simulink model "V_F_Control_induction_motor"  (R2017a)
settings: Solver=ode23t  StartTime=0.0  StopTime=10  FixedStep=1e-6  RelTol=1e-3
libraries: powerlib x10, simulink x3
settings Model: SimulationMode=accelerator  Creator=Aslam  LastModifiedBy=Administrator
settings DataIOCC: SaveFormat=StructureWithTime
settings OptimizationCC: LifeSpan=inf
settings DebuggingCC: SFExecutionAtInitializationDiag=none
settings HardwareCC: ProdBitPerSizeT=32  ProdBitPerPtrDiffT=32  ProdWordSize=32  ProdHWDeviceType=Specified

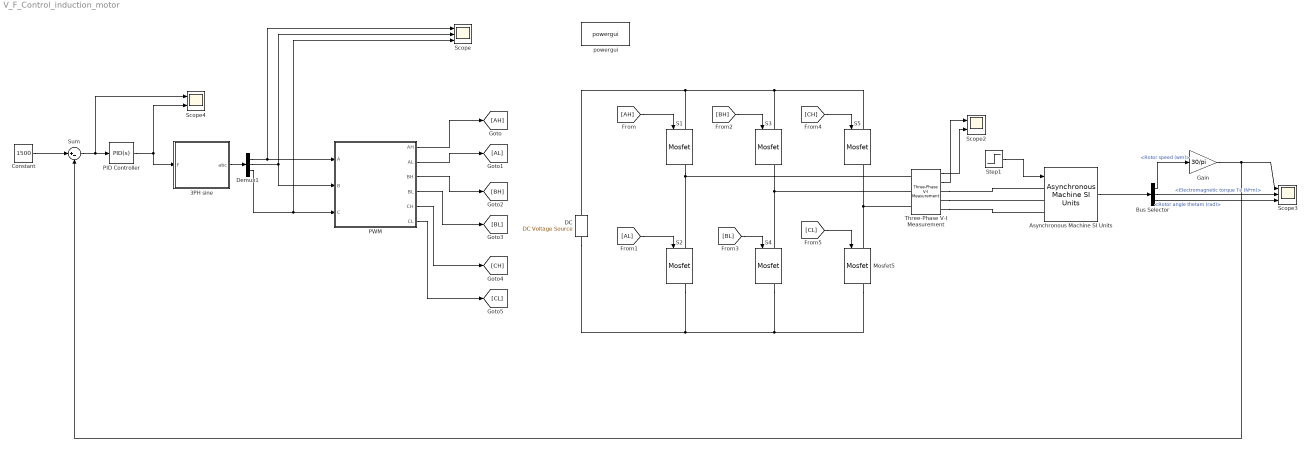
== system V_F_Control_induction_motor ==
  3PH sine : Subsystem
  Asynchronous Machine SI Units : powerlib/Machines/Asynchronous Machine SI Units  RotorType=Squirrel-cage  PresetModel="01:  5 HP   460 V 60Hz 1750 RPM"  MechanicalLoad=Torque Tm  ShowDetailedParameters=on  ReferenceFrame=Rotor  Units=SI  MeasurementBus=off  NominalParameters=[3730 460 60]  Stator=[1.115 0.005974]  Rotor=[1.083 0.005974]  Cage1=[0.4155 0.002066]  Cage2=[0.4168 0.0003495]  Lm=0.2037  Mechanical=[0.02 0.005752 2]  PolePairs=2  InitialConditions=[0 0 0 0 0 0 0 0]  SimulateSaturation=off  Saturation=[14.03593122, 27.81365428, 53.79336849, 72.68890987, 97.98006896, 148.6815601, 215.7428561, 302.9841135, 428.7778367 ; 230, 322, 414, 460, 506, 552, 598, 644, 690]  LoadFlowParameters=1492000  TsPowergui=0  TsBlock=-1  IterativeModel=Trapezoidal non iterative  IterativeDiscreteModel=Trapezoidal non iterative  Pmec=1.492e+006
  Bus Selector : BusSelector  OutputSignals=Mechanical.Rotor speed (wm),Mechanical.Electromagnetic torque Te (N*m),Mechanical.Rotor angle thetam (rad)
  Constant : Constant  Value=1500
  DC : powerlib/Electrical Sources/DC Voltage Source  Amplitude=600  Measurements=None
  Demux1 : Demux  Outputs=3
  Gain : Gain  Gain=30/pi
  Mosfet5 : powerlib/Power Electronics/Mosfet  Ron=0.1  Lon=0  Rd=0.01  Vfd=0  IC=0  Rs=1e5  Cs=inf  Measurements=on
  PID Controller : simulink/Continuous/PID Controller  Controller=PID  TimeDomain=Continuous-time  SampleTime=-1  IntegratorMethod=Forward Euler  FilterMethod=Forward Euler  Form=Parallel  UseFilter=on  ControllerParametersSource=internal  P=0.01  I=0.1  D=0  N=100  InitialConditionSource=internal  InitialConditionForIntegrator=0  InitialConditionForFilter=0  ExternalReset=none  LimitOutput=off  UpperSaturationLimit=inf  LowerSaturationLimit=-inf  LinearizeAsGain=on  AntiWindupMode=none  Kb=1  TrackingMode=off  Kt=1  PParamMin=[]  PParamMax=[]  IParamMin=[]  IParamMax=[]  DParamMin=[]  DParamMax=[]  NParamMin=[]  NParamMax=[]  KbParamMin=[]  KbParamMax=[]  KtParamMin=[]  KtParamMax=[]  POutMin=[]  POutMax=[]  IOutMin=[]  IOutMax=[]  DOutMin=[]  DOutMax=[]  NOutMin=[]  NOutMax=[]  KbOutMin=[]  KbOutMax=[]  KtOutMin=[]  KtOutMax=[]  IntegratorOutMin=[]  IntegratorOutMax=[]  FilterOutMin=[]  FilterOutMax=[]  SumOutMin=[]  SumOutMax=[]  SumI1OutMin=[]  SumI1OutMax=[]  SumI2OutMin=[]  SumI2OutMax=[]  SumI3OutMin=[]  SumI3OutMax=[]  SumDOutMin=[]  SumDOutMax=[]  SaturationOutMin=[]  SaturationOutMax=[]  IntegratorContinuousStateAttributes=''  IntegratorStateMustResolveToSignalObject=off  IntegratorRTWStateStorageClass=Auto  FilterContinuousStateAttributes=''  FilterStateMustResolveToSignalObject=off  FilterRTWStateStorageClass=Auto  DifferentiatorICPrevScaledInput=0  DifferentiatorOutMin=[]  DifferentiatorOutMax=[]  InitialConditionSetting=State (most efficient)
  PWM : Subsystem
  S{1..5} (5 alike) : powerlib/Power Electronics/Mosfet  Ron=0.1  Lon=0  Rd=0.01  Vfd=0  IC=0  Rs=1e5  Cs=inf  Measurements=on
  Scope : Scope  NumInputPorts=3
  Scope2 : Scope  NumInputPorts=2
  Scope3 : Scope  NumInputPorts=3
  Scope4 : Scope  NumInputPorts=2
  Step1 : Step  Time=5  Before=5  After=10  SampleTime=0
  Sum : Sum  Inputs=|+-
  Three-Phase V-I Measurement : powerlib/Measurements/Three-Phase V-I Measurement  VoltageMeasurement=phase-to-phase  SetLabelV=off  LabelV=Vabc  Vpu=off  VpuLL=off  CurrentMeasurement=yes  SetLabelI=off  LabelI=Iabc  Ipu=off  Pbase=100e6  Vbase=500e3  OutputType=Complex  PhasorSimulation=off  PSBequivalent=0
  powergui : powerlib/powergui  Priority=1  SimulationMode=Discrete  SampleTime=10e-6  frequency=60  Iterations=50  frequencyindice=0  Pbase=100e6  ErrMax=1e-4  UnitsV=kV  UnitsW=MW  buscounter=0  FunctionMessages=off  echomessages=off  EnableUseOfTLC=off  CurrentSourceSwitches=off  DisableSnubberDevices=off  DisableRonSwitches=off  DisableVfSwitches=off  DisplayEquations=off  SolverType=Tustin/Backward Euler (TBE)  Interpol=off  ExternalGateDelay=off  methode=off  Ts=100  x0status=blocks  SPID=off  SwTol=0  HookPort=off  RestoreLinks=warning  ResistiveCurrentMeasurement=off  Frange=[0:2:500]  Ylog=off  Xlog=on  ShowGrid=off  save=off  variable=ZData  structure=0  ZoomFFT=off  StartTime=0.0  cycles=1  DisplayStyle=1  fundamental=60  FreqAxis=off  MaxFrequency=1000  frequencyindicesteady=1  RmsSteady=1  display=off
  wires:
  Demux1/1 -> Scope/1, PWM/1(A)
  Demux1/2 -> Scope/2, PWM/2(B)
  Demux1/3 -> Scope/3, PWM/3(C)
  PWM/1(AH) -> [AH]
  PWM/2(AL) -> [AL]
  PWM/3(BH) -> [BH]
  PWM/4(BL) -> [BL]
  PWM/5(CH) -> [CH]
  PWM/6(CL) -> [CL]
  [AH] -> S1/1
  [AL] -> S2/1
  [BH] -> S3/1
  [BL] -> S4/1
  [CH] -> S5/1
  [CL] -> Mosfet5/1
  Three-Phase V-I Measurement/2 -> Scope2/1
  Three-Phase V-I Measurement/1 -> Scope2/2
  Asynchronous Machine SI Units/1 -> Bus Selector/1
  Bus Selector/1 -> Gain/1  "<Rotor speed (wm)>"
  Bus Selector/2 -> Scope3/2  "<Electromagnetic torque Te (N*m)>"
  Bus Selector/3 -> Scope3/3  "<Rotor angle thetam (rad)>"
  Gain/1 -> Sum/2, Scope3/1
  Sum/1 -> Scope4/1, PID Controller/1
  Constant/1 -> Sum/1
  PID Controller/1 -> 3PH sine/1(F), Scope4/2
  3PH sine/1(abc) -> Demux1/1
  Step1/1 -> Asynchronous Machine SI Units/1
  connections:
  DC/RConn1 -- S5/LConn1 -- S3/LConn1 -- S1/LConn1
  DC/LConn1 -- S2/RConn1 -- Mosfet5/RConn1 -- S4/RConn1
  Mosfet5/LConn1 -- Three-Phase V-I Measurement/LConn3 -- S5/RConn1
  S4/LConn1 -- Three-Phase V-I Measurement/LConn2 -- S3/RConn1
  S1/RConn1 -- S2/LConn1 -- Three-Phase V-I Measurement/LConn1
  Three-Phase V-I Measurement/RConn1 -- Asynchronous Machine SI Units/LConn1
  Three-Phase V-I Measurement/RConn2 -- Asynchronous Machine SI Units/LConn2
  Three-Phase V-I Measurement/RConn3 -- Asynchronous Machine SI Units/LConn3

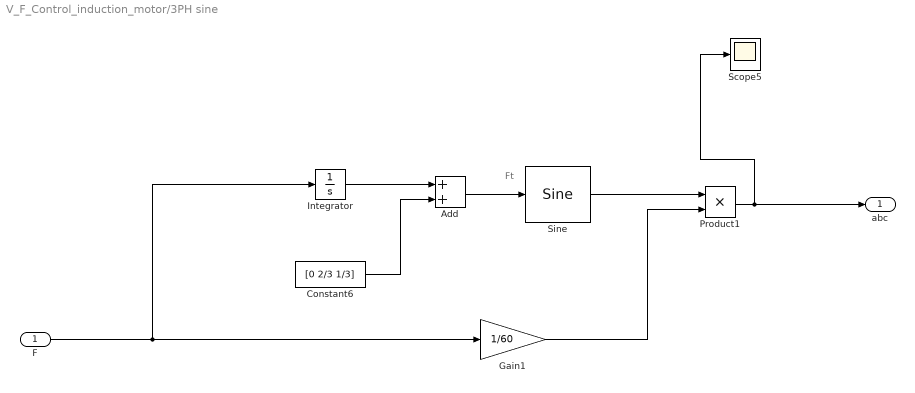
== system V_F_Control_induction_motor/3PH sine ==
  note: Ft
  F : Inport
  Add : Sum
  Constant6 : Constant  Value=[0 2/3 1/3]
  Gain1 : Gain  Gain=1/60
  Integrator : Integrator
  Product1 : Product
  Scope5 : Scope
  Sine : simulink/Lookup Tables/Sine  Formula=sin(2*pi*u)  NumDataPoints=(2^5)+1  OutputWordLength=16  InternalRulePriority=Speed
      settings: SourceProductName=Simulink
  abc : Outport
  wires:
  F/1 -> Gain1/1, Integrator/1
  Gain1/1 -> Product1/2
  Sine/1 -> Product1/1
  Product1/1 -> abc/1, Scope5/1
  Constant6/1 -> Add/2
  Add/1 -> Sine/1
  Integrator/1 -> Add/1

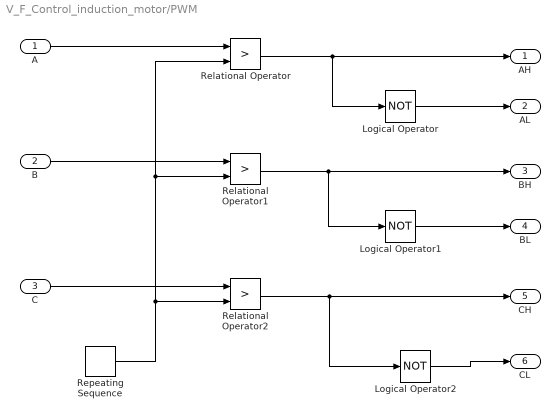
== system V_F_Control_induction_motor/PWM ==
  A : Inport
  B : Inport  Port=2
  C : Inport  Port=3
  Logical Operator : Logic  Operator=NOT  IconShape=distinctive  AllPortsSameDT=off  OutDataTypeStr=boolean
  Logical Operator1 : Logic  Operator=NOT  IconShape=distinctive  AllPortsSameDT=off  OutDataTypeStr=boolean
  Logical Operator2 : Logic  Operator=NOT  IconShape=distinctive  AllPortsSameDT=off  OutDataTypeStr=boolean
  Relational Operator : RelationalOperator  Operator=>  OutDataTypeStr=boolean  RndMeth=Nearest
  Relational Operator1 : RelationalOperator  Operator=>  OutDataTypeStr=boolean  RndMeth=Nearest
  Relational Operator2 : RelationalOperator  Operator=>  OutDataTypeStr=boolean  RndMeth=Nearest
  Repeating Sequence : simulink/Sources/Repeating Sequence  rep_seq_t=[0 0.5/5000 1/5000]  rep_seq_y=[-1 1 -1]
  AH : Outport
  AL : Outport  Port=2
  BH : Outport  Port=3
  BL : Outport  Port=4
  CH : Outport  Port=5
  CL : Outport  Port=6
  wires:
  A/1 -> Relational Operator/1
  C/1 -> Relational Operator2/1
  Repeating Sequence/1 -> Relational Operator1/2, Relational Operator/2, Relational Operator2/2
  B/1 -> Relational Operator1/1
  Relational Operator/1 -> Logical Operator/1, AH/1
  Logical Operator/1 -> AL/1
  Relational Operator1/1 -> Logical Operator1/1, BH/1
  Logical Operator1/1 -> BL/1
  Relational Operator2/1 -> CH/1, Logical Operator2/1
  Logical Operator2/1 -> CL/1
